simulink model "simulink_ROS_subscribers"  (R2019b)
settings: Solver=FixedStepAuto  StartTime=0.0  StopTime=Inf  FixedStep=FIXED_STEP_SIZE  RelTol=1e-3
undefined symbols (not defined in the file): RAD2DEG
libraries: robotlib x4
settings Model: Creator=ananda  LastModifiedBy=ananda

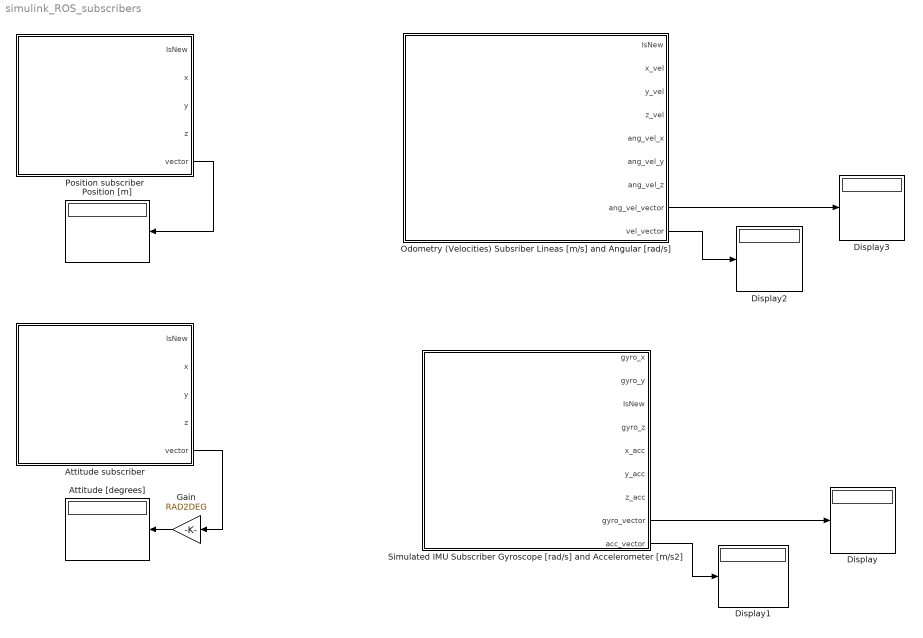
== system simulink_ROS_subscribers ==
  Attitude [degrees] : Display
  Attitude subscriber : Subsystem
  Display{,1..3} (4 alike) : Display
  Gain : Gain  Gain=RAD2DEG
  Odometry (Velocities) Subsriber Lineas [m/s] and Angular [rad/s] : Subsystem
  Position [m] : Display
  Position subscriber : Subsystem
  Simulated IMU Subscriber Gyroscope [rad/s] and Accelerometer [m/s2] : Subsystem
  wires:
  Position subscriber/5(vector) -> Position [m]/1
  Gain/1 -> Attitude [degrees]/1
  Attitude subscriber/5(vector) -> Gain/1
  Simulated IMU Subscriber Gyroscope [rad/s] and Accelerometer [m/s2]/8(gyro_vector) -> Display/1
  Simulated IMU Subscriber Gyroscope [rad/s] and Accelerometer [m/s2]/9(acc_vector) -> Display1/1
  Odometry (Velocities) Subsriber Lineas [m/s] and Angular [rad/s]/9(vel_vector) -> Display2/1
  Odometry (Velocities) Subsriber Lineas [m/s] and Angular [rad/s]/8(ang_vel_vector) -> Display3/1

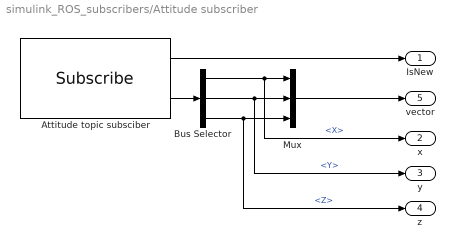
== system simulink_ROS_subscribers/Attitude subscriber ==
  Attitude topic subsciber : robotlib/Subscribe  topicSource=Specify your own  topic=/ardrone/orientation_rpy  messageType=geometry_msgs/Vector3  sampleTime=ATTI_SUB_DT  messageQueueLength=1
      settings: SourceProductName=ROS Toolbox
  Bus Selector : BusSelector  OutputSignals=X,Y,Z
  Mux : Mux  Inputs=3
  IsNew : Outport
  x : Outport  Port=2
  y : Outport  Port=3
  z : Outport  Port=4
  vector : Outport  Port=5
  wires:
  Bus Selector/3 -> z/1, Mux/3  "<Z>"
  Bus Selector/2 -> y/1, Mux/2  "<Y>"
  Bus Selector/1 -> x/1, Mux/1  "<X>"
  Attitude topic subsciber/2 -> Bus Selector/1
  Attitude topic subsciber/1 -> IsNew/1
  Mux/1 -> vector/1

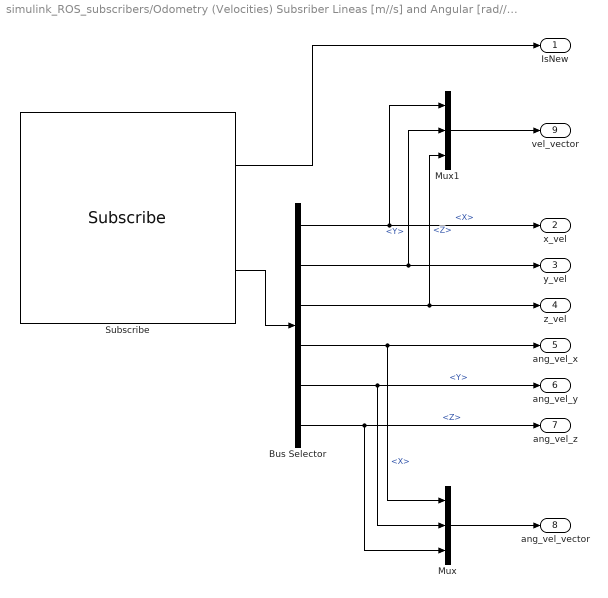
== system simulink_ROS_subscribers/Odometry (Velocities) Subsriber Lineas [m//s] and Angular [rad//s] ==
  Bus Selector : BusSelector  OutputSignals=Twist.Twist.Linear.X,Twist.Twist.Linear.Y,Twist.Twist.Linear.Z,Twist.Twist.Angular.X,Twist.Twist.Angular.Y,Twist.Twist.Angular.Z
  Mux : Mux  Inputs=3
  Mux1 : Mux  Inputs=3
  Subscribe : robotlib/Subscribe  topicSource=Specify your own  topic=/ardrone/odometry_sensor1/odometry  messageType=nav_msgs/Odometry  sampleTime=ODOMETRY_SUB_DT  messageQueueLength=1
      settings: SourceProductName=ROS Toolbox
  IsNew : Outport
  x_vel : Outport  Port=2
  y_vel : Outport  Port=3
  z_vel : Outport  Port=4
  ang_vel_x : Outport  Port=5
  ang_vel_y : Outport  Port=6
  ang_vel_z : Outport  Port=7
  ang_vel_vector : Outport  Port=8
  vel_vector : Outport  Port=9
  wires:
  Bus Selector/4 -> Mux/1, ang_vel_x/1  "<X>"
  Bus Selector/6 -> Mux/3, ang_vel_z/1  "<Z>"
  Bus Selector/2 -> Mux1/2, y_vel/1  "<Y>"
  Subscribe/1 -> IsNew/1
  Bus Selector/5 -> Mux/2, ang_vel_y/1  "<Y>"
  Bus Selector/1 -> Mux1/1, x_vel/1  "<X>"
  Subscribe/2 -> Bus Selector/1
  Bus Selector/3 -> Mux1/3, z_vel/1  "<Z>"
  Mux/1 -> ang_vel_vector/1
  Mux1/1 -> vel_vector/1

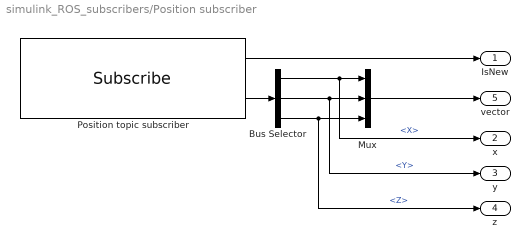
== system simulink_ROS_subscribers/Position subscriber ==
  Bus Selector : BusSelector  OutputSignals=Point.X,Point.Y,Point.Z
  Mux : Mux  Inputs=3
  Position topic subscriber : robotlib/Subscribe  topicSource=Specify your own  topic=/ardrone/odometry_sensor1/position  messageType=geometry_msgs/PointStamped  sampleTime=POS_SUB_DT  messageQueueLength=1
      settings: SourceProductName=ROS Toolbox
  IsNew : Outport
  x : Outport  Port=2
  y : Outport  Port=3
  z : Outport  Port=4
  vector : Outport  Port=5
  wires:
  Bus Selector/3 -> z/1, Mux/3  "<Z>"
  Bus Selector/2 -> y/1, Mux/2  "<Y>"
  Mux/1 -> vector/1
  Bus Selector/1 -> x/1, Mux/1  "<X>"
  Position topic subscriber/2 -> Bus Selector/1
  Position topic subscriber/1 -> IsNew/1

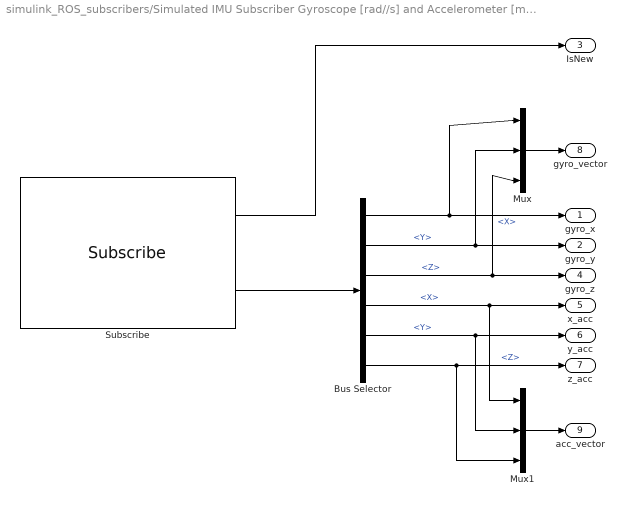
== system simulink_ROS_subscribers/Simulated IMU Subscriber Gyroscope [rad//s] and Accelerometer [m//s2] ==
  Bus Selector : BusSelector  OutputSignals=AngularVelocity.X,AngularVelocity.Y,AngularVelocity.Z,LinearAcceleration.X,LinearAcceleration.Y,LinearAcceleration.Z
  Mux : Mux  Inputs=3
  Mux1 : Mux  Inputs=3
  Subscribe : robotlib/Subscribe  topicSource=Specify your own  topic=/ardrone/imu  messageType=sensor_msgs/Imu  sampleTime=IMU_SUB_DT  messageQueueLength=1
      settings: SourceProductName=ROS Toolbox
  gyro_x : Outport
  gyro_y : Outport  Port=2
  IsNew : Outport  Port=3
  gyro_z : Outport  Port=4
  x_acc : Outport  Port=5
  y_acc : Outport  Port=6
  z_acc : Outport  Port=7
  gyro_vector : Outport  Port=8
  acc_vector : Outport  Port=9
  wires:
  Bus Selector/6 -> Mux1/3, z_acc/1  "<Z>"
  Bus Selector/2 -> Mux/2, gyro_y/1  "<Y>"
  Bus Selector/5 -> Mux1/2, y_acc/1  "<Y>"
  Subscribe/2 -> Bus Selector/1
  Subscribe/1 -> IsNew/1
  Bus Selector/4 -> Mux1/1, x_acc/1  "<X>"
  Bus Selector/3 -> Mux/3, gyro_z/1  "<Z>"
  Bus Selector/1 -> Mux/1, gyro_x/1  "<X>"
  Mux/1 -> gyro_vector/1
  Mux1/1 -> acc_vector/1
